simulink model "dlb_sm2022b"  (R2022b)
settings: Solver=FixedStepAuto  StartTime=0.0  StopTime=10.0  FixedStep=1e-6  RelTol=1e-3
settings Model: Creator=Zenos  LastModifiedBy=Zenos
settings OptimizationCC: ReuseModelBlockBuffer=on

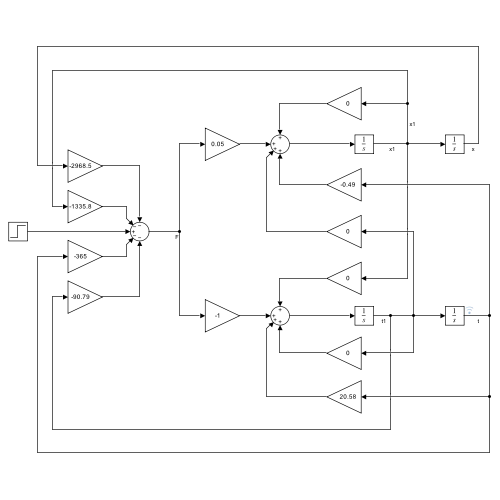
[thumbnail: Simulink's stored preview of the top-level diagram]
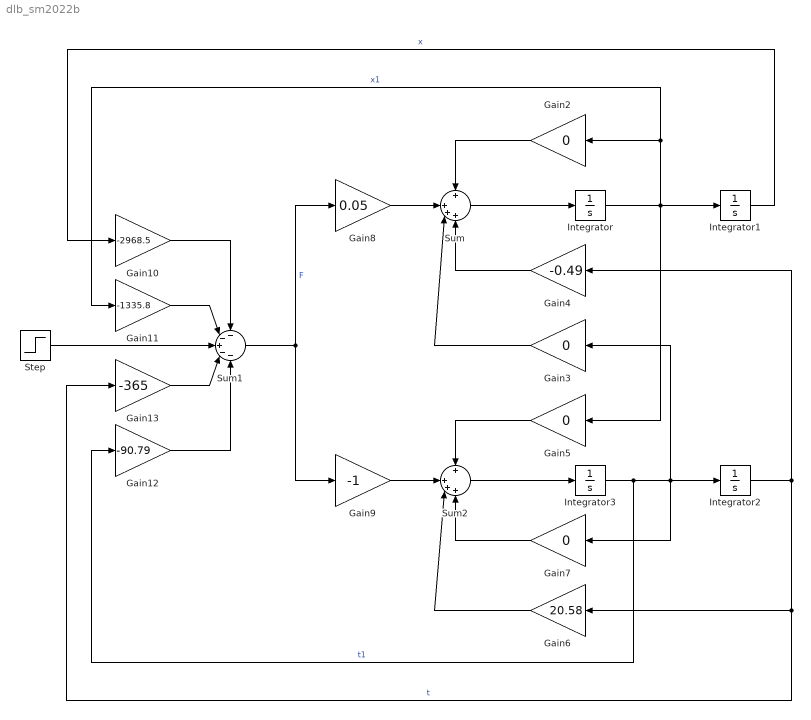
== system dlb_sm2022b ==
  Gain10 : Gain  Gain=-2968.5
  Gain11 : Gain  Gain=-1335.8
  Gain12 : Gain  Gain=-90.79
  Gain13 : Gain  Gain=-365
  Gain{2..3,5,7} (4 alike) : Gain  Gain=0
  Gain4 : Gain  Gain=-0.49
  Gain6 : Gain  Gain=20.58
  Gain8 : Gain  Gain=0.05
  Gain9 : Gain  Gain=-1
  Integrator : Integrator
  Integrator1 : Integrator
  Integrator2 : Integrator  InitialCondition=-1
  Integrator3 : Integrator
  Step : Step  After=1000  SampleTime=0
  Sum : Sum  Inputs=+|+++
  Sum1 : Sum  Inputs=--+--
  Sum2 : Sum  Inputs=+|+++
  wires:
  Integrator/1 -> Gain11/1, Gain2/1, Gain5/1, Integrator1/1  "x1"
  Integrator3/1 -> Gain7/1, Integrator2/1, Gain3/1, Gain12/1  "t1"
  Integrator2/1 -> Gain6/1, Gain13/1, Gain4/1  "t"
  Sum/1 -> Integrator/1
  Gain2/1 -> Sum/1
  Gain3/1 -> Sum/3
  Gain4/1 -> Sum/4
  Gain5/1 -> Sum2/1
  Sum2/1 -> Integrator3/1
  Gain6/1 -> Sum2/3
  Gain7/1 -> Sum2/4
  Gain8/1 -> Sum/2
  Gain9/1 -> Sum2/2
  Sum1/1 -> Gain9/1, Gain8/1  "F"
  Integrator1/1 -> Gain10/1  "x"
  Gain10/1 -> Sum1/1
  Gain11/1 -> Sum1/2
  Gain13/1 -> Sum1/4
  Gain12/1 -> Sum1/5
  Step/1 -> Sum1/3
